simulink model "asbCubeSatACS"  (R2025b)
settings: Solver=FixedStepDiscrete  StartTime=0.0  StopTime=1000  FixedStep=CubeSatTimeStep  RelTol=1e-3  EnableMultiTasking=on
undefined symbols (not defined in the file): gains
libraries: slpidlib x3, aerolibutil x2, sharedtransform x2, aerolibsatdyn x1
settings Model: DataDictionary=asbCubeSatModelData.sldd  ExtModeAutoUpdateStatusClock=off  Creator=The MathWorks, Inc.  LastModifiedBy=alokahn
settings SolverCC: AlgebraicLoopSolver=TrustRegion  MaxZcPerStep=1.0
settings DataIOCC: LimitDataPoints=on  SaveFormat=Array  SaveOutput=off  SignalLogging=off  DSMLogging=off  SaveTime=off  ReturnWorkspaceOutputs=off
settings OptimizationCC: DefaultParameterBehavior=Inlined  OptimizeBlockIOStorage=off  BufferReuse=off  GlobalBufferReuse=off  ExpressionFolding=off  ExpressionDepthLimit=2147483647.0  LocalBlockOutputs=off  InitFltsAndDblsToZero=on  LifeSpan=inf  OptimizeDataStoreBuffers=off  BusAssignmentInplaceUpdate=off
settings DebuggingCC: ArtificialAlgebraicLoopMsg=none  SolverPrmCheckMsg=warning  FcnCallInpInsideContextMsg=warning  UnconnectedInputMsg=warning  UnconnectedOutputMsg=warning  UnconnectedLineMsg=warning  StateNameClashWarn=warning  PregeneratedLibrarySubsystemCodeDiagnostic=none  SFUnexpectedBacktrackingDiag=warning  SFNoUnconditionalDefaultTransitionDiag=warning  SFExecutionAtInitializationDiag=none  ArithmeticOperatorsInVariantConditions=warning
settings HardwareCC: ProdBitPerPointer=32.0  ProdBitPerSizeT=32.0  ProdBitPerPtrDiffT=32.0  ProdLargestAtomicFloat=None  ProdIntDivRoundTo=Undefined  ProdEndianess=Unspecified  ProdWordSize=32.0  ProdHWDeviceType=32-bit Generic
settings ModelReferenceCC: EnableRefExpFcnMdlSchedulingChecks=on  PropagateSignalLabelsOutOfModel=off
settings SFSimCC: SimUseLocalCustomCode=off
settings RTWCC: RTWUseLocalCustomCode=off  GPUComputeCapability=3.5  DLArmComputeVersion=19.05
settings CodeAppCC: StateflowObjectComments=on
settings GRTTargetCC: TargetFcnLib=ansi_tfl_tmw.mat  TargetLangStandard=C89/C90 (ANSI)  CombineOutputUpdateFcns=off  GRTInterface=on
settings ConfigComp: CovMetricSettings=dw  CovSaveCumulativeToWorkspaceVar=on  CovSaveSingleToWorkspaceVar=on  CovExternalEMLEnable=off

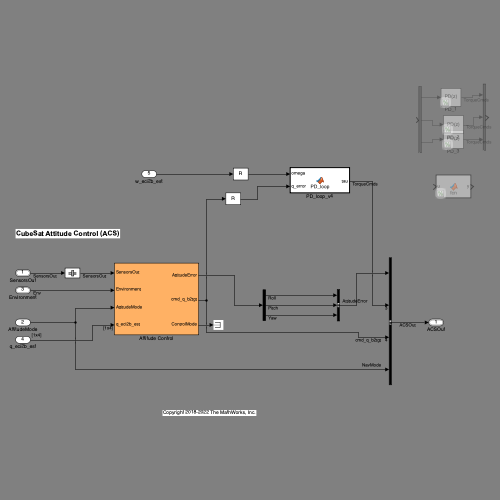
[thumbnail: Simulink's stored preview of the top-level diagram]
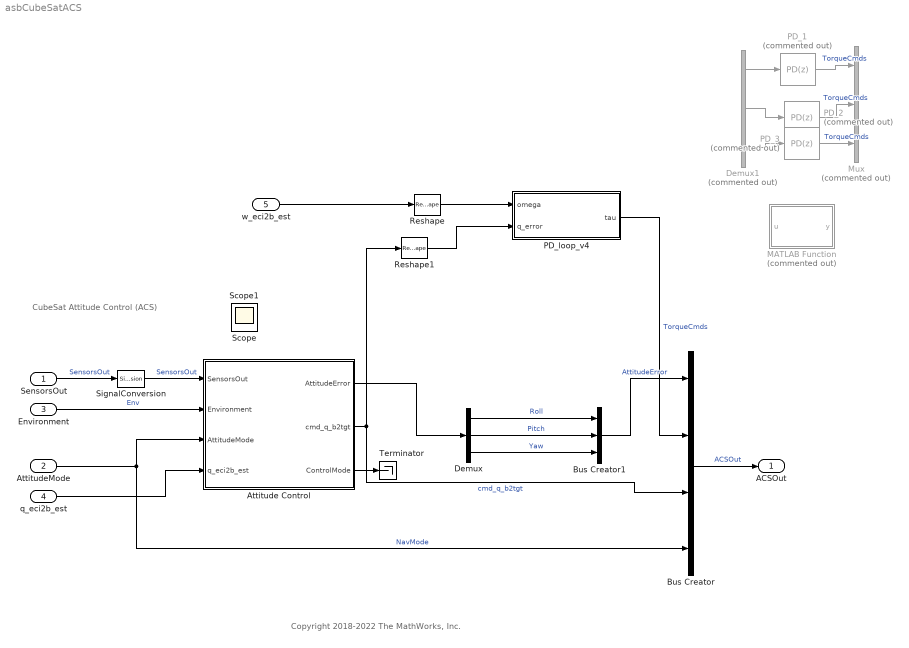
== system asbCubeSatACS ==
  note: Copyright 2018-2022 The MathWorks, Inc.
  note: CubeSat Attitude Control (ACS)
  SensorsOut : Inport  OutDataTypeStr=Bus: StatesOutBus
  AttitudeMode : Inport  Port=2  OutDataTypeStr=double  PortDimensions=1
  Environment : Inport  Port=3  OutDataTypeStr=Bus: EnvBus  PortDimensions=1
  q_eci2b_est : Inport  Port=4  PortDimensions=[1,4]  SampleTime=1
  w_eci2b_est : Inport  Port=5  SampleTime=1
  Attitude Control : Subsystem
  Bus Creator : BusCreator  Inputs=4  OutDataTypeStr=Bus: ACSOutBus  NonVirtualBus=on
  Bus Creator1 : BusCreator  Inputs=3  OutDataTypeStr=Bus: AttitudeErrorBus
  Demux : Demux  Outputs=3
  Demux1 : Demux  Commented=on  Outputs=3
  MATLAB Function : MATLAB Function  Commented=on  TreatAsAtomicUnit=on
  Mux : Mux  Commented=on  Inputs=3
  PD_1 : slpidlib/PID Controller  Commented=on  Controller=PD  Form=Parallel  TimeDomain=Discrete-time  UseExternalTs=off  SampleTime=-1  IntegratorMethod=Forward Euler  FilterMethod=Forward Euler  ControllerParametersSource=internal  P=0.0098  I=gains.Ki  UseKiTs=off  D=0.0240  UseExternalDerivativeSource=off  N=1000  UseFilter=off  TunerSelectOption=Frequency Response Based  InitialConditionSource=internal  InitialConditionForIntegrator=0  InitialConditionForFilter=0  DifferentiatorICPrevScaledInput=0  ExternalReset=none  TrackingMode=off  Kt=1  LimitOutput=off  SatLimitsSource=internal  UpperSaturationLimit=inf  LowerSaturationLimit=-inf  LinearizeAsGain=off  AntiWindupMode=none  Kb=1  LimitIntegrator=off  UpperIntegratorSaturationLimit=inf  LowerIntegratorSaturationLimit=-inf  POutMin=[]  POutMax=[]  IOutMin=[]  IOutMax=[]  DOutMin=[]  DOutMax=[]  NOutMin=[]  NOutMax=[]  SumOutMin=[]  SumOutMax=[]  SaturationOutMin=[]  SaturationOutMax=[]  PParamMin=[]  PParamMax=[]  IParamMin=[]  IParamMax=[]  DParamMin=[]  DParamMax=[]  NParamMin=[]  NParamMax=[]  KbParamMin=[]  KbParamMax=[]  KtParamMin=[]  KtParamMax=[]  KbOutMin=[]  KbOutMax=[]  KtOutMin=[]  KtOutMax=[]  IntegratorOutMin=[]  IntegratorOutMax=[]  FilterOutMin=[]  FilterOutMax=[]  SumI1OutMin=[]  SumI1OutMax=[]  SumI2OutMin=[]  SumI2OutMax=[]  SumI3OutMin=[]  SumI3OutMax=[]  SumI4OutMin=[]  SumI4OutMax=[]  SumDOutMin=[]  SumDOutMax=[]  DifferentiatorOutMin=[]  DifferentiatorOutMax=[]  FilterDiffOutCoefMin=[]  FilterDiffOutCoefMax=[]  ReciprocalOutMin=[]  ReciprocalOutMax=[]  SumDenOutMin=[]  SumDenOutMax=[]  SumNumOutMin=[]  SumNumOutMax=[]  DivideOutMin=[]  DivideOutMax=[]  UdiffTsProdOutMin=[]  UdiffTsProdOutMax=[]  NTsProdOutMin=[]  NTsProdOutMax=[]  UintegralTsProdOutMin=[]  UintegralTsProdOutMax=[]  UngainTsProdOutMin=[]  UngainTsProdOutMax=[]  ClampingZeroOutDataTypeStr=Inherit: Inherit via back propagation  ClampingZeroOutMin=[]  ClampingZeroOutMax=[]  FilterDenConstantOutDataTypeStr=Inherit: Inherit via back propagation  FilterDenConstantOutMin=[]  FilterDenConstantOutMax=[]  PCopyOutDataTypeStr=Inherit: Inherit via back propagation  PCopyOutMin=[]  PCopyOutMax=[]  NCopyOutDataTypeStr=Inherit: Inherit via back propagation  NCopyOutMin=[]  NCopyOutMax=[]  IntegratorContinuousStateAttributes=''  IntegratorStateMustResolveToSignalObject=off  IntegratorRTWStateStorageClass=Auto  FilterContinuousStateAttributes=''  FilterStateMustResolveToSignalObject=off  FilterRTWStateStorageClass=Auto  ParallelPVariant=InternalParameters  IdealPVariant=Disabled  IVariant=Disabled  DVariant=InternalParameters  IntegratorVariant=Disabled  SatVariant=Disabled  AWVariant=Disabled  PCopyVariant=Disabled  TRVariant=Disabled  FdbkBlocksVariant=Forward  IdealPFdbkVariant=Disabled  SatFdbkVariant=Disabled  DerivativeFilterVariant=Differentiator  NVariant=Passthrough  NCopyVariant=Disabled_SignalSpec  FilterICVariant=InternalICsDifferentiator  IntegratorICVariant=Disabled  ExternalResetVariant=Disabled  TRSumVariant=Passthrough  SumFdbkVariant=Disabled  SumVariant=Sum_PD  TsampFilterVariant=InternalTs  TsampNgainVariant=Passthrough  TsampIntegralVariant=Disabled_SignalSpec  ExternalSaturationOutDataTypeStr=Inherit: Same as second input  DerivativeSourceVariant=ErrorSignal  PreIntVariant=InternalPreInt
  PD_2 : slpidlib/PID Controller  Commented=on  Controller=PD  Form=Parallel  TimeDomain=Discrete-time  UseExternalTs=off  SampleTime=-1  IntegratorMethod=Forward Euler  FilterMethod=Forward Euler  ControllerParametersSource=internal  P=0.0082  I=gains.Ki  UseKiTs=off  D=0.0200  UseExternalDerivativeSource=off  N=1000  UseFilter=off  TunerSelectOption=Frequency Response Based  InitialConditionSource=internal  InitialConditionForIntegrator=0  InitialConditionForFilter=0  DifferentiatorICPrevScaledInput=0  ExternalReset=none  TrackingMode=off  Kt=1  LimitOutput=off  SatLimitsSource=internal  UpperSaturationLimit=inf  LowerSaturationLimit=-inf  LinearizeAsGain=off  AntiWindupMode=none  Kb=1  LimitIntegrator=off  UpperIntegratorSaturationLimit=inf  LowerIntegratorSaturationLimit=-inf  POutMin=[]  POutMax=[]  IOutMin=[]  IOutMax=[]  DOutMin=[]  DOutMax=[]  NOutMin=[]  NOutMax=[]  SumOutMin=[]  SumOutMax=[]  SaturationOutMin=[]  SaturationOutMax=[]  PParamMin=[]  PParamMax=[]  IParamMin=[]  IParamMax=[]  DParamMin=[]  DParamMax=[]  NParamMin=[]  NParamMax=[]  KbParamMin=[]  KbParamMax=[]  KtParamMin=[]  KtParamMax=[]  KbOutMin=[]  KbOutMax=[]  KtOutMin=[]  KtOutMax=[]  IntegratorOutMin=[]  IntegratorOutMax=[]  FilterOutMin=[]  FilterOutMax=[]  SumI1OutMin=[]  SumI1OutMax=[]  SumI2OutMin=[]  SumI2OutMax=[]  SumI3OutMin=[]  SumI3OutMax=[]  SumI4OutMin=[]  SumI4OutMax=[]  SumDOutMin=[]  SumDOutMax=[]  DifferentiatorOutMin=[]  DifferentiatorOutMax=[]  FilterDiffOutCoefMin=[]  FilterDiffOutCoefMax=[]  ReciprocalOutMin=[]  ReciprocalOutMax=[]  SumDenOutMin=[]  SumDenOutMax=[]  SumNumOutMin=[]  SumNumOutMax=[]  DivideOutMin=[]  DivideOutMax=[]  UdiffTsProdOutMin=[]  UdiffTsProdOutMax=[]  NTsProdOutMin=[]  NTsProdOutMax=[]  UintegralTsProdOutMin=[]  UintegralTsProdOutMax=[]  UngainTsProdOutMin=[]  UngainTsProdOutMax=[]  ClampingZeroOutDataTypeStr=Inherit: Inherit via back propagation  ClampingZeroOutMin=[]  ClampingZeroOutMax=[]  FilterDenConstantOutDataTypeStr=Inherit: Inherit via back propagation  FilterDenConstantOutMin=[]  FilterDenConstantOutMax=[]  PCopyOutDataTypeStr=Inherit: Inherit via back propagation  PCopyOutMin=[]  PCopyOutMax=[]  NCopyOutDataTypeStr=Inherit: Inherit via back propagation  NCopyOutMin=[]  NCopyOutMax=[]  IntegratorContinuousStateAttributes=''  IntegratorStateMustResolveToSignalObject=off  IntegratorRTWStateStorageClass=Auto  FilterContinuousStateAttributes=''  FilterStateMustResolveToSignalObject=off  FilterRTWStateStorageClass=Auto  ParallelPVariant=InternalParameters  IdealPVariant=Disabled  IVariant=Disabled  DVariant=InternalParameters  IntegratorVariant=Disabled  SatVariant=Disabled  AWVariant=Disabled  PCopyVariant=Disabled  TRVariant=Disabled  FdbkBlocksVariant=Forward  IdealPFdbkVariant=Disabled  SatFdbkVariant=Disabled  DerivativeFilterVariant=Differentiator  NVariant=Passthrough  NCopyVariant=Disabled_SignalSpec  FilterICVariant=InternalICsDifferentiator  IntegratorICVariant=Disabled  ExternalResetVariant=Disabled  TRSumVariant=Passthrough  SumFdbkVariant=Disabled  SumVariant=Sum_PD  TsampFilterVariant=InternalTs  TsampNgainVariant=Passthrough  TsampIntegralVariant=Disabled_SignalSpec  ExternalSaturationOutDataTypeStr=Inherit: Same as second input  DerivativeSourceVariant=ErrorSignal  PreIntVariant=InternalPreInt
  PD_3 : slpidlib/PID Controller  Commented=on  Controller=PD  Form=Parallel  TimeDomain=Discrete-time  UseExternalTs=off  SampleTime=-1  IntegratorMethod=Forward Euler  FilterMethod=Forward Euler  ControllerParametersSource=internal  P=0.0031  I=gains.Ki  UseKiTs=off  D=0.0076  UseExternalDerivativeSource=off  N=1000  UseFilter=off  TunerSelectOption=Transfer Function Based (PID Tuner App)  InitialConditionSource=internal  InitialConditionForIntegrator=0  InitialConditionForFilter=0  DifferentiatorICPrevScaledInput=0  ExternalReset=none  TrackingMode=off  Kt=1  LimitOutput=off  SatLimitsSource=internal  UpperSaturationLimit=inf  LowerSaturationLimit=-inf  LinearizeAsGain=off  AntiWindupMode=none  Kb=1  LimitIntegrator=off  UpperIntegratorSaturationLimit=inf  LowerIntegratorSaturationLimit=-inf  POutMin=[]  POutMax=[]  IOutMin=[]  IOutMax=[]  DOutMin=[]  DOutMax=[]  NOutMin=[]  NOutMax=[]  SumOutMin=[]  SumOutMax=[]  SaturationOutMin=[]  SaturationOutMax=[]  PParamMin=[]  PParamMax=[]  IParamMin=[]  IParamMax=[]  DParamMin=[]  DParamMax=[]  NParamMin=[]  NParamMax=[]  KbParamMin=[]  KbParamMax=[]  KtParamMin=[]  KtParamMax=[]  KbOutMin=[]  KbOutMax=[]  KtOutMin=[]  KtOutMax=[]  IntegratorOutMin=[]  IntegratorOutMax=[]  FilterOutMin=[]  FilterOutMax=[]  SumI1OutMin=[]  SumI1OutMax=[]  SumI2OutMin=[]  SumI2OutMax=[]  SumI3OutMin=[]  SumI3OutMax=[]  SumI4OutMin=[]  SumI4OutMax=[]  SumDOutMin=[]  SumDOutMax=[]  DifferentiatorOutMin=[]  DifferentiatorOutMax=[]  FilterDiffOutCoefMin=[]  FilterDiffOutCoefMax=[]  ReciprocalOutMin=[]  ReciprocalOutMax=[]  SumDenOutMin=[]  SumDenOutMax=[]  SumNumOutMin=[]  SumNumOutMax=[]  DivideOutMin=[]  DivideOutMax=[]  UdiffTsProdOutMin=[]  UdiffTsProdOutMax=[]  NTsProdOutMin=[]  NTsProdOutMax=[]  UintegralTsProdOutMin=[]  UintegralTsProdOutMax=[]  UngainTsProdOutMin=[]  UngainTsProdOutMax=[]  ClampingZeroOutDataTypeStr=Inherit: Inherit via back propagation  ClampingZeroOutMin=[]  ClampingZeroOutMax=[]  FilterDenConstantOutDataTypeStr=Inherit: Inherit via back propagation  FilterDenConstantOutMin=[]  FilterDenConstantOutMax=[]  PCopyOutDataTypeStr=Inherit: Inherit via back propagation  PCopyOutMin=[]  PCopyOutMax=[]  NCopyOutDataTypeStr=Inherit: Inherit via back propagation  NCopyOutMin=[]  NCopyOutMax=[]  IntegratorContinuousStateAttributes=''  IntegratorStateMustResolveToSignalObject=off  IntegratorRTWStateStorageClass=Auto  FilterContinuousStateAttributes=''  FilterStateMustResolveToSignalObject=off  FilterRTWStateStorageClass=Auto  ParallelPVariant=InternalParameters  IdealPVariant=Disabled  IVariant=Disabled  DVariant=InternalParameters  IntegratorVariant=Disabled  SatVariant=Disabled  AWVariant=Disabled  PCopyVariant=Disabled  TRVariant=Disabled  FdbkBlocksVariant=Forward  IdealPFdbkVariant=Disabled  SatFdbkVariant=Disabled  DerivativeFilterVariant=Differentiator  NVariant=Passthrough  NCopyVariant=Disabled_SignalSpec  FilterICVariant=InternalICsDifferentiator  IntegratorICVariant=Disabled  ExternalResetVariant=Disabled  TRSumVariant=Passthrough  SumFdbkVariant=Disabled  SumVariant=Sum_PD  TsampFilterVariant=InternalTs  TsampNgainVariant=Passthrough  TsampIntegralVariant=Disabled_SignalSpec  ExternalSaturationOutDataTypeStr=Inherit: Same as second input  DerivativeSourceVariant=ErrorSignal  PreIntVariant=InternalPreInt
  PD_loop_v4 : MATLAB Function  TreatAsAtomicUnit=on  SystemSampleTime=1
  Reshape : Reshape  OutputDimensionality=Customize  OutputDimensions=[3,1]
  Reshape1 : Reshape  OutputDimensionality=Customize  OutputDimensions=[4, 1]
  SignalConversion : SignalConversion  ConversionOutput=Virtual bus  OverrideOpt=off
  Terminator : Terminator
  ACSOut : Outport  OutDataTypeStr=Bus: ACSOutBus  PortDimensions=1  VectorParamsAs1DForOutWhenUnconnected=off  BusOutputAsStruct=on
  Scope : Scope
  Scope1 : Scope
      settings: ActiveDisplayYMinimum=-0.13646382044925889  ActiveDisplayYMaximum=3.23106670458966
  wires:
  Demux/1 -> Bus Creator1/1  "Roll"
  AttitudeMode/1 -> Bus Creator/4, Attitude Control/3("AttitudeMode ")  "NavMode"
  Demux/2 -> Bus Creator1/2  "Pitch"
  SensorsOut/1 -> SignalConversion/1  "SensorsOut"
  Bus Creator1/1 -> Bus Creator/1  "AttitudeError"
  Demux/3 -> Bus Creator1/3  "Yaw"
  Bus Creator/1 -> ACSOut/1  "ACSOut"
  Attitude Control/3(" ControlMode") -> Terminator/1
  Environment/1 -> Attitude Control/2(Environment)  "Env"
  Attitude Control/2(cmd_q_b2tgt) -> Reshape1/1, Bus Creator/3  "cmd_q_b2tgt"
  SignalConversion/1 -> Attitude Control/1("SensorsOut ")  "SensorsOut"
  Demux1/3 -> PD_3/1
  PD_3/1 -> Mux/3  "TorqueCmds"
  PD_2/1 -> Mux/2  "TorqueCmds"
  Demux1/2 -> PD_2/1
  Reshape/1 -> PD_loop_v4/1(omega)
  Attitude Control/1(AttitudeError) -> Demux/1
  PD_1/1 -> Mux/1  "TorqueCmds"
  Demux1/1 -> PD_1/1
  PD_loop_v4/1(tau) -> Bus Creator/2  "TorqueCmds"
  Reshape1/1 -> PD_loop_v4/2(q_error)
  q_eci2b_est/1 -> Attitude Control/4(q_eci2b_est)
  w_eci2b_est/1 -> Reshape/1

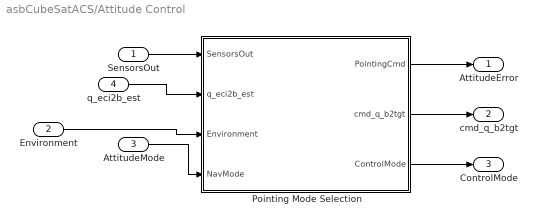
== system asbCubeSatACS/Attitude Control ==
  "SensorsOut " : Inport  OutDataTypeStr=Bus: StatesOutBus
  Environment : Inport  Port=2
  "AttitudeMode " : Inport  Port=3
  q_eci2b_est : Inport  Port=4  PortDimensions=[1,4]
  Pointing Mode Selection : Stateflow chart  RequirementInfo="{}  %GIDa_a065c7c8_537d_4123_b3cc_6e7e7008a32c"  TreatAsAtomicUnit=on
  AttitudeError : Outport  VectorParamsAs1DForOutWhenUnconnected=off
  cmd_q_b2tgt : Outport  Port=2  VectorParamsAs1DForOutWhenUnconnected=off
  " ControlMode" : Outport  Port=3  VectorParamsAs1DForOutWhenUnconnected=off
  wires:
  "SensorsOut "/1 -> Pointing Mode Selection/1(SensorsOut)
  Pointing Mode Selection/3(ControlMode) -> " ControlMode"/1
  "AttitudeMode "/1 -> Pointing Mode Selection/4(NavMode)
  Environment/1 -> Pointing Mode Selection/3(Environment)
  Pointing Mode Selection/1(PointingCmd) -> AttitudeError/1
  Pointing Mode Selection/2(cmd_q_b2tgt) -> cmd_q_b2tgt/1
  q_eci2b_est/1 -> Pointing Mode Selection/2(q_eci2b_est)

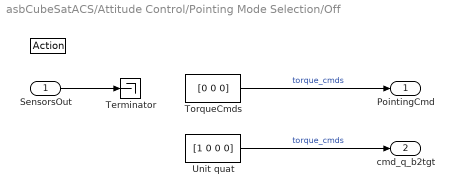
== system asbCubeSatACS/Attitude Control/Pointing Mode Selection/Off ==
  SensorsOut : Inport  OutDataTypeStr=Bus: StatesOutBus
  " " : ActionPort
      settings: CopyFcn=Stateflow.SLINSF.SimulinkMan.removeBlockPreDeleteFcn  PreDeleteFcn=Stateflow.SLINSF.SimulinkMan.unsafePredeleteFcn
  Terminator : Terminator
  TorqueCmds : Constant  Value=[0 0 0]
  Unit quat : Constant  Value=[1 0 0 0]
  PointingCmd : Outport  RequirementInfo="{}  %GIDa_4dc055f9_6cac_42e1_8ddb_4145586b89f5"  VectorParamsAs1DForOutWhenUnconnected=off
  cmd_q_b2tgt : Outport  RequirementInfo="{}  %GIDa_ca05d0a6_a581_4c3e_b3a0_cd281b586de8"  Port=2  VectorParamsAs1DForOutWhenUnconnected=off
  wires:
  SensorsOut/1 -> Terminator/1
  TorqueCmds/1 -> PointingCmd/1  "torque_cmds"
  Unit quat/1 -> cmd_q_b2tgt/1  "torque_cmds"

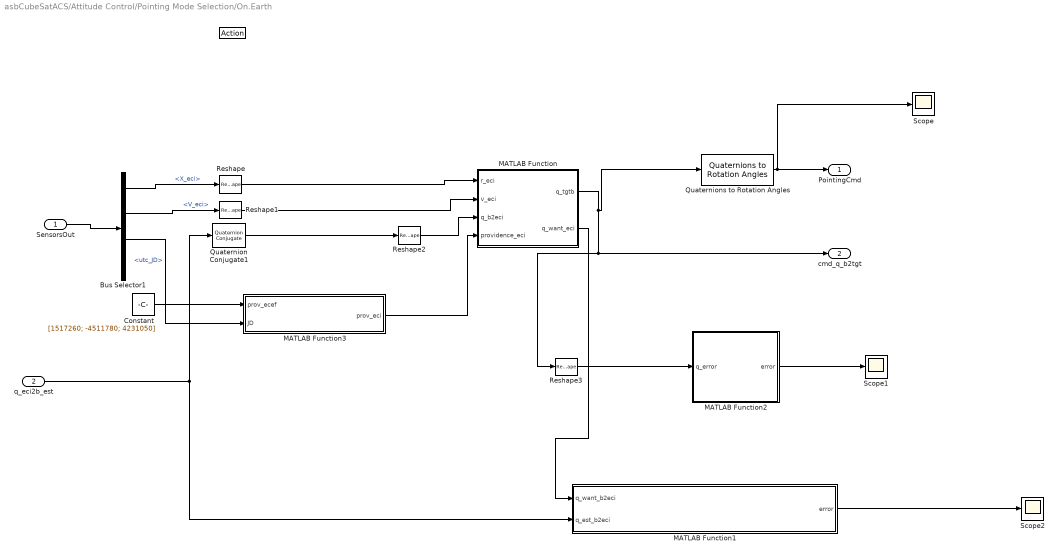
== system asbCubeSatACS/Attitude Control/Pointing Mode Selection/On.Earth ==
  SensorsOut : Inport  OutDataTypeStr=Bus: StatesOutBus
  q_eci2b_est : Inport  Port=2  PortDimensions=[1,4]
  " " : ActionPort
      settings: CopyFcn=Stateflow.SLINSF.SimulinkMan.removeBlockPreDeleteFcn  PreDeleteFcn=Stateflow.SLINSF.SimulinkMan.unsafePredeleteFcn
  Bus Selector1 : BusSelector  OutputSignals=X_eci,V_eci,utc_JD,q_eci2b
  Constant : Constant  Value=[1517260; -4511780; 4231050]
  MATLAB Function : MATLAB Function  TreatAsAtomicUnit=on
  MATLAB Function1 : MATLAB Function  TreatAsAtomicUnit=on
  MATLAB Function2 : MATLAB Function  TreatAsAtomicUnit=on
  MATLAB Function3 : MATLAB Function  TreatAsAtomicUnit=on
  Quaternion Conjugate1 : aerolibutil/Quaternion Conjugate
  Quaternions to Rotation Angles : sharedtransform/Quaternions to Rotation Angles  rotationOrder=XYZ  aMode=aMode
  Reshape : Reshape  OutputDimensionality=Column vector (2-D)
  Reshape1 : Reshape  OutputDimensionality=Column vector (2-D)
  Reshape2 : Reshape  OutputDimensionality=Customize  OutputDimensions=[1,4]
  Reshape3 : Reshape  OutputDimensionality=Customize  OutputDimensions=[1,4]
  Scope : Scope
      settings: ActiveDisplayYMinimum=-1.0198327701548264  ActiveDisplayYMaximum=2.2885054349185885  DataLoggingVariableName=ScopeData2
  Scope1 : Scope
      settings: ActiveDisplayYMinimum=-0.082257069515711156  ActiveDisplayYMaximum=0.20936508608070933  DataLoggingVariableName=ScopeData3
  Scope2 : Scope
      settings: ActiveDisplayYMinimum=-0.082257069515711156  ActiveDisplayYMaximum=0.20936508608070933  DataLoggingVariableName=ScopeData4
  PointingCmd : Outport  VectorParamsAs1DForOutWhenUnconnected=off
  cmd_q_b2tgt : Outport  RequirementInfo="{}  %GIDa_69a01501_0b6a_41cf_b570_f5b49bb229cd"  Port=2  VectorParamsAs1DForOutWhenUnconnected=off
  wires:
  Quaternions to Rotation Angles/1 -> Scope/1, PointingCmd/1
  SensorsOut/1 -> Bus Selector1/1
  Bus Selector1/2 -> Reshape1/1  "<V_eci>"
  Bus Selector1/1 -> Reshape/1  "<X_eci>"
  Quaternion Conjugate1/1 -> Reshape2/1
  Reshape/1 -> MATLAB Function/1(r_eci)
  Reshape1/1 -> MATLAB Function/2(v_eci)
  Reshape2/1 -> MATLAB Function/3(q_b2eci)
  MATLAB Function/1(q_tgtb) -> Quaternions to Rotation Angles/1, Reshape3/1, cmd_q_b2tgt/1
  MATLAB Function2/1(error) -> Scope1/1
  Reshape3/1 -> MATLAB Function2/1(q_error)
  Bus Selector1/3 -> MATLAB Function3/2(JD)  "<utc_JD>"
  Constant/1 -> MATLAB Function3/1(prov_ecef)
  MATLAB Function3/1(prov_eci) -> MATLAB Function/4(providence_eci)
  MATLAB Function/2(q_want_eci) -> MATLAB Function1/1(q_want_b2eci)
  q_eci2b_est/1 -> Quaternion Conjugate1/1, MATLAB Function1/2(q_est_b2eci)
  MATLAB Function1/1(error) -> Scope2/1

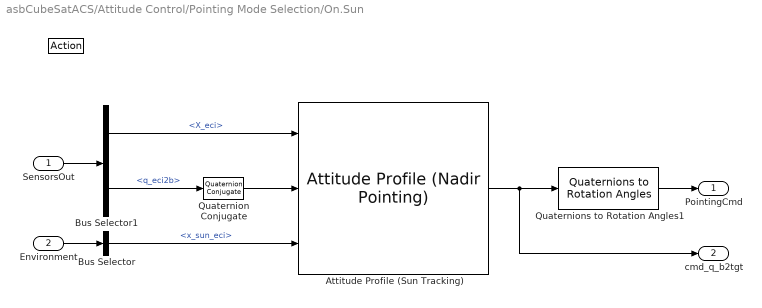
== system asbCubeSatACS/Attitude Control/Pointing Mode Selection/On.Sun ==
  SensorsOut : Inport  OutDataTypeStr=Bus: StatesOutBus
  Environment : Inport  Port=2  OutDataTypeStr=Bus: EnvBus
  " " : ActionPort
      settings: CopyFcn=Stateflow.SLINSF.SimulinkMan.removeBlockPreDeleteFcn  PreDeleteFcn=Stateflow.SLINSF.SimulinkMan.unsafePredeleteFcn
  Attitude Profile (Sun Tracking) : aerolibsatdyn/Attitude Profile (Nadir Pointing)  outputError=on  outputFinalAttitude=off  portFrame=ICRF  pointingMode=Custom  celestialTarget=Sun  tunablePointing=off  primaryAlignmentSrc=Dialog  primaryAlignment=[0 0 -1]  secondaryAlignmentSrc=Dialog  secondaryAlignment=[1 0 0]  constraintFrame=ICRF  primaryConstraintSrc=Port  primaryConstraint=[1 0 0]  secondaryConstraintSrc=Dialog  secondaryConstraint=[0 0 1]
  Bus Selector : BusSelector  OutputSignals=x_sun_eci
  Bus Selector1 : BusSelector  OutputSignals=X_eci,q_eci2b
  Quaternion Conjugate : aerolibutil/Quaternion Conjugate
  Quaternions to Rotation Angles1 : sharedtransform/Quaternions to Rotation Angles  rotationOrder=XYZ  aMode=aMode
  PointingCmd : Outport  VectorParamsAs1DForOutWhenUnconnected=off
  cmd_q_b2tgt : Outport  Port=2  VectorParamsAs1DForOutWhenUnconnected=off
  wires:
  Attitude Profile (Sun Tracking)/1 -> Quaternions to Rotation Angles1/1, cmd_q_b2tgt/1
  SensorsOut/1 -> Bus Selector1/1
  Environment/1 -> Bus Selector/1
  Quaternions to Rotation Angles1/1 -> PointingCmd/1
  Bus Selector/1 -> Attitude Profile (Sun Tracking)/3  "<x_sun_eci>"
  Quaternion Conjugate/1 -> Attitude Profile (Sun Tracking)/2
  Bus Selector1/2 -> Quaternion Conjugate/1  "<q_eci2b>"
  Bus Selector1/1 -> Attitude Profile (Sun Tracking)/1  "<X_eci>"

== matlab function asbCubeSatACS/MATLAB Function ==
  data: u input; y output
function y = fcn(u)
    y = u;
end

% --- OVERVIEW: 
% {vec(q_want), vec(q_current), vec(q_omega)} ->
% {vec(tau)} ->
% {vec(m)} (magnetic moment)

% Given 3 quaternions, {q_want, q_expected, q_omega}, return the torque needed at
% that time

function [m] = get_m(q_want, q_current, r_omega, B)
    arguments
        q_want (4,1) double
        q_current (4,1) double 
        r_omega (1,4) double % angular velocity in axis-angle format (gyro)
        B (1,3) double % magnetic field (x, y, z)
    end
    e = error_axis_angle(q_want, q_current);
    m = PD_loop(e, r_omega, B);
end

function [m] = tau_to_m(tau, B)
% Obtains wanted magnetic moment from wanted torque and current magnetic field
    arguments
        tau (1,3) double % torque (x, y, z)
        B (1,3) double % magnetic field (x, y, z)
        end
    m = cross(B, tau) / (norm(B)^2);
end

function [e] = error_axis_angle(q_want, q_current)
% Obtains r_e, the error vector in axis-angle format
    arguments
        q_want (1,4) double 
        q_current (1,4) double 
    end
    q_error = quatmultiply(q_want, quatinv(q_current));
    angle = 2 * acos(q_error(1));
    axis = q_error(2:4) / sin(angle/2); 
    
    e = [axis; angle];
end

function [tau] = PD_loop(r_e, r_omega)
    arguments
        r_e (4,1) double % axis-angle error vector
        r_omega (4,1) double % angular velocity in axis-angle format (gyro)
    end
    Kp0 = 5.5 * 10^(-5);
    Kd0 = 0.017;
    Kp = [Kp0, Kp0, Kp0]; % (to be changed) 
    Kd = [Kd0, Kd0, Kd0]; % (to be changed)

    tau = zeros(3, 1);

    for i = 1:3
        Pi = Kp(i) * r_e(4) * r_e(i);
        Di = Kd(i) * r_omega(4) * r_omega(i);
        tau(i) = Pi + Di;
    end
end

function [m] = PD_loop_m(r_e, r_omega, B)
    arguments
        r_e (4,1) double % axis-angle error vector
        r_omega (4,1) double % angular velocity in axis-angle format (gyro)
        B (3,1) double % Magnetic field vector (x, y, z)
    end
    placeholder = 1;
    Kp = [-placeholder, -placeholder, -placeholder]; % (to be changed) 
    Kd = [-placeholder, -placeholder, -placeholder]; % (to be changed)

    tau = zeros(3, 1);

    for i = 1:3
        Pi = Kp(i) * r_e(4) * r_e(i);
        Di = Kd(i) * r_omega(4) * r_omega(i);
        tau(i) = Pi + Di;
    end

    m = tau_to_m(tau, B);
end

== matlab function asbCubeSatACS/Attitude Control/Pointing Mode Selection/On.Earth/MATLAB Function1 ==
  data: q_want_b2eci input; error output; q_est_b2eci input
function error = fcn(q_want_b2eci, q_est_b2eci)
    q_error = quat_multiply(quatinv(q_want_b2eci), q_est_b2eci);
    if q_error(1) < 0
        q_error = -q_error;
    end
    error = 2 * acos(q_error(1));
    rad2deg(error);
end

== matlab function asbCubeSatACS/Attitude Control/Pointing Mode Selection/On.Earth/MATLAB Function2 ==
  data: q_error input; error output
function error = fcn(q_error)
    if q_error(1) < 0
        q_error = -q_error;
    end
    error = 2 * acos(q_error(1));
    rad2deg(error);
end

== matlab function asbCubeSatACS/PD_loop_v4 ==
  data: omega input; q_error input; tau output
% INPUTS:
% omega - (3 x 1), deg/s: w_eci2b in body coordinates, that is angular velocity wr/ to eci
% written in body coordinates
% q_error - (4 x 1): error quaternion from pointing_error, scalar first

% RETURN:
% tau - torque in N-m, body coordinates


function tau = PD_loop(omega, q_error)

    arguments
        omega (3,1) double
        q_error (4, 1) double
    end
    %find shortest possible rotation
    if (q_error(1) < 0)
        q_error = -q_error;
    end

   
    angle = 2 * acos(q_error(1));

    if angle > 1e-12
        axis = q_error(2:4) / sin(angle/2);
    else
        axis = [0; 0; 0];
    end
    r_e = [axis; angle];
    % Convert 3x1 error omega vector back to axis-angle
    omega_rad = omega * (pi/180); % omega is in deg/s. converting to rad/s
    omega_mag = norm(omega_rad);
   
    if omega_mag > 1e-12
        omega_axis = omega_rad / omega_mag;
    else
        omega_axis = [0; 0; 0];
    end
    
    r_omega = [omega_axis; omega_mag];

    % PD controller
    Kp0 = 0.034;
    Kd0 = 0.42;
    max_tau = 5;
    I_body = [3.0054115e-02, -5.1674000e-05, 2.5075000e-05 ;-5.1674000e-05, 1.1430611e-02, -3.6481690e-03 ;2.5075000e-05, -3.6481690e-03, 2.3052295e-02];
    
    Kp = [Kp0, Kp0, Kp0];
    Kd = [Kd0, Kd0, Kd0];
    tau = zeros(3,1);

    for i = 1:3
        Pi = Kp(i) * r_e(4) * r_e(i);
        Di = Kd(i) * r_omega(4) * r_omega(i);
        tau(i) = Pi - Di;
    end
    tau = I_body * tau;
    tau = min(tau, max_tau);
end

== matlab function asbCubeSatACS/Attitude Control/Pointing Mode Selection/On.Earth/MATLAB Function3 ==
  data: prov_ecef input; prov_eci output; JD input
function prov_eci = eceftoeci(prov_ecef, JD)
    % Step 1: Unix time -> Julian Date

    % Step 2: Julian Date -> GMST (degrees)
    theta_deg = jd_to_gmst(JD);

    % Step 3: Build rotation matrix R_z(theta)
    theta = deg2rad(theta_deg);
    R = [ cos(theta), -sin(theta), 0; ...
          sin(theta),  cos(theta), 0; ...
          0,           0,          1];

    % Step 4: Rotate position
    prov_eci = R * prov_ecef;

end


% -------------------------------------------------------------------------
function theta_deg = jd_to_gmst(JD)
% JD_TO_GMST Compute Greenwich Mean Sidereal Time (degrees) from Julian Date.

    % Julian centuries since J2000.0
    T = (JD - 2451545.0) / 36525.0;

    % GMST in degrees
    theta_deg = 280.46061837 ...
              + 360.98564736629 * (JD - 2451545.0) ...
              + 0.000387933     * T^2 ...
              - T^3             / 38710000.0;

    % Reduce to [0, 360)
    theta_deg = mod(theta_deg, 360.0);
end

== stateflow chart asbCubeSatACS/Attitude Control/Pointing Mode Selection ==
  state On
    state Transition
    state Earth
    state Sun
    (default) -> Transition
    Transition -> Sun [order 2] : [NavMode == 2]
        | {ControlMode = 2;}
    Sun -> Transition : [NavMode == 1]
        | {ControlMode = 1;}
    Transition -> Earth [order 1] : [NavMode == 1]
        | {ControlMode = 2;}
    Earth -> Transition : [NavMode == 2]
        | {ControlMode = 1;}
  state Off
  (default) -> Off
  Off -> On : [NavMode ~= 0]
      | {ControlMode = 1;}
  On -> Off : [NavMode == 0]
      | {ControlMode = 0;}
  data: sf_internal_action_state_placeholder_data local double size=1 =0; sf_internal_action_state_placeholder_data local double size=1 =0; sf_internal_action_state_placeholder_data local double size=1 =0; SensorsOut input Bus: StatesOutBus; q_eci2b_est input; Environment input; NavMode input; PointingCmd output =[0 0 0]'; cmd_q_b2tgt output; ControlMode output

== matlab function asbCubeSatACS/Attitude Control/Pointing Mode Selection/On.Earth/MATLAB Function ==
  data: r_eci input; q_tgtb output; v_eci input; q_b2eci input; providence_eci input; q_want_eci output
% INPUTS:
% r_eci - (3 x 1): ECI coordinates of satellite position
% v_eci - (3 x 1): ECI velocity of sattelite position
% q_b2eci - (1 x 4): quaternion of current orientation in ECI to BODY frame
% providence_eci - (1 x 3): ECI coordinates of Providence, Rhode Island
%
% RETURN:
% q_tgtb - (1 x 4): error quaternion, with axis in body coordinates
%
function [q_tgtb, q_want_eci] = pointing_error(r_eci, v_eci, q_b2eci, providence_eci)
    
    providence_eci = [0; 0; 0];
    persistent q_want_prev 
    if isempty(q_want_prev)
        q_want_prev = [1 0 0 0];   % initial guess, any unit quaternion
    end
    z_want = providence_eci - r_eci;
    z_want = z_want / norm(z_want);

    y_want = cross(z_want, v_eci);
    y_want = y_want / norm(y_want);

    x_want = cross(y_want, z_want);
    x_want = x_want / norm(x_want);

    R_want_eci = [x_want, y_want, z_want];

    q_want_eci = rotm2quat(R_want_eci);
    if dot(q_want_eci, q_want_prev) < 0
        q_want_eci = -q_want_eci;
    end
    q_want_prev = q_want_eci;   % store for next timestep
   
    q_tgtb = quatmultiply(q_b2eci, q_want_eci);
  
end
